simulink model "Temporal1NoActions"  (Simulink 9.0)
settings: Solver=ode45  StartTime=0.0  StopTime=20  RelTol=1e-3  EnableMultiTasking=on
settings Model: SuppressorTable=22 serialization::archive 11 0 6 0 0 0 0 0  Creator=scaife  LastModifiedBy=ktrinh  ExtModeAutoUpdateStatusClock=off
settings DataIOCC: LimitDataPoints=on  SignalLoggingSaveFormat=ModelDataLogs  SignalLoggingName=sigsOut
settings DebuggingCC: SaveWithParameterizedLinksMsg=none  SignalResolutionControl=TryResolveAllWithWarning  MultiTaskDSMMsg=warning  MultiTaskCondExecSysMsg=none
settings HardwareCC: TargetUnknown=on
settings SFSimCC: SimParseCustomCode=off
settings GRTTargetCC: CombineOutputUpdateFcns=off  GRTInterface=on

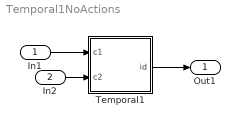
== system Temporal1NoActions ==
  In1 : Inport  OutDataTypeStr=boolean
  In2 : Inport  Port=2  OutDataTypeStr=boolean
  Temporal1 : Stateflow chart  TreatAsAtomicUnit=on
  Out1 : Outport
  wires:
  Temporal1/1(id) -> Out1/1
  In1/1 -> Temporal1/1(c1)
  In2/1 -> Temporal1/2(c2)

== stateflow chart Temporal1 ==
  state A/
    en : id=2;
  state B/
    en : id=1;
  (default) -> A
  A -> B : [c1]
  B -> A : [c2]
  data: c1 input double; c2 input double; id output double
